simulink model "example1"  (R2024b)
settings: Solver=FixedStepAuto  StartTime=0.0  StopTime=20  FixedStep=0.001  RelTol=1e-3
(part 3 of 3)

== system example1/Subsystem15/SAT ==
  In1 : Inport
  Constant : Constant  Value=-1000
  Constant1 : Constant  Value=1000
  If : If  IfExpression=u1 < -1000  ElseIfExpressions=u1 > 1000
  If Action Subsystem : Subsystem  TreatAsAtomicUnit=on
  If Action Subsystem1 : Subsystem  TreatAsAtomicUnit=on
  If Action Subsystem2 : Subsystem  TreatAsAtomicUnit=on
  Merge : Merge  Inputs=3
  u1 : Outport
  wires:
  In1/1 -> If Action Subsystem1/1(In1), If/1
  If/1 -> If Action Subsystem/Action
  Constant/1 -> If Action Subsystem/1(In1)
  If/3 -> If Action Subsystem1/Action
  If/2 -> If Action Subsystem2/Action
  Constant1/1 -> If Action Subsystem2/1(In1)
  If Action Subsystem/1(Out1) -> Merge/1
  If Action Subsystem1/1(Out1) -> Merge/3
  If Action Subsystem2/1(Out1) -> Merge/2
  Merge/1 -> u1/1

== system example1/Subsystem15/Subsystem ==
  alpha : Inport
  Abs : Abs  SaturateOnIntegerOverflow=off
  Abs1 : Abs  SaturateOnIntegerOverflow=off
  Add : Sum  Inputs=+-
  Constant : Constant  Value=1/2
  Constant1 : Constant  Value=2/3
  Divide : Product  Inputs=*/
  Gain : Gain  Gain=-1
  Integrator : Integrator
  Integrator1 : Integrator
  Pow : Math  Operator=pow  SignedPower=on  RndMeth=Zero
  Pow1 : Math  Operator=pow  SignedPower=on  RndMeth=Zero
  Product{,1..3} (4 alike) : Product
  Product4 : Product  Inputs=3
  Sign : Signum
  Sign1 : Signum
  Sum : Sum  Inputs=|++
  k1 : Constant  Value=0.01
  k2 : Constant  Value=0.1
  xi : Constant
  tao1 : Outport
  tao2 : Outport  Port=2
  wires:
  alpha/1 -> Add/2
  Add/1 -> Pow/1, Sign/1
  Constant/1 -> Pow/2
  Pow/1 -> Abs/1
  Abs/1 -> Product/2
  Sign/1 -> Product/1
  Product/1 -> Product1/2
  k1/1 -> Product1/1
  Product1/1 -> Sum/1
  xi/1 -> Product4/2, Product4/3, Divide/2
  Divide/1 -> Sign1/1, Pow1/1
  Constant1/1 -> Pow1/2
  Pow1/1 -> Abs1/1
  Abs1/1 -> Product2/2
  Sign1/1 -> Product2/1
  Product2/1 -> Product3/1
  k2/1 -> Product3/2
  Product3/1 -> Sum/2
  Sum/1 -> Product4/1
  Product4/1 -> Gain/1
  Gain/1 -> Integrator/1
  Integrator/1 -> Divide/1, Integrator1/1, tao2/1
  Integrator1/1 -> Add/1, tao1/1

== system example1/Subsystem15/g22 ==
  x21 : Inport
  x22 : Inport  Port=2
  Constant : Constant  Value=4/5
  Sin : Trigonometry
  Sum : Sum  Inputs=|++
  Sum1 : Sum  Inputs=|++
  "[2]^1_1" : Subsystem
  g22 : Outport
  wires:
  x22/1 -> Sum1/2, "[2]^1_1"/2(2)
  Constant/1 -> "[2]^1_1"/1(In1)
  "[2]^1_1"/1(Out1) -> Sum/2
  Sum/1 -> g22/1
  x21/1 -> Sum1/1
  Sum1/1 -> Sin/1
  Sin/1 -> Sum/1

== system example1/Subsystem17/SAT ==
  In1 : Inport
  Constant : Constant  Value=-2000
  Constant1 : Constant  Value=2000
  If : If  IfExpression=u1 < -2000  ElseIfExpressions=u1 > 2000
  If Action Subsystem : Subsystem  TreatAsAtomicUnit=on
  If Action Subsystem1 : Subsystem  TreatAsAtomicUnit=on
  If Action Subsystem2 : Subsystem  TreatAsAtomicUnit=on
  Merge : Merge  Inputs=3
  u1 : Outport
  wires:
  In1/1 -> If Action Subsystem1/1(In1), If/1
  If/1 -> If Action Subsystem/Action
  Constant/1 -> If Action Subsystem/1(In1)
  If/3 -> If Action Subsystem1/Action
  If/2 -> If Action Subsystem2/Action
  Constant1/1 -> If Action Subsystem2/1(In1)
  If Action Subsystem/1(Out1) -> Merge/1
  If Action Subsystem1/1(Out1) -> Merge/3
  If Action Subsystem2/1(Out1) -> Merge/2
  Merge/1 -> u1/1

== system example1/Subsystem17/Subsystem ==
  alpha : Inport
  Abs : Abs  SaturateOnIntegerOverflow=off
  Abs1 : Abs  SaturateOnIntegerOverflow=off
  Add : Sum  Inputs=+-
  Constant : Constant  Value=1/2
  Constant1 : Constant  Value=2/3
  Divide : Product  Inputs=*/
  Gain : Gain  Gain=-1
  Integrator : Integrator
  Integrator1 : Integrator
  Pow : Math  Operator=pow  SignedPower=on  RndMeth=Zero
  Pow1 : Math  Operator=pow  SignedPower=on  RndMeth=Zero
  Product{,1..3} (4 alike) : Product
  Product4 : Product  Inputs=3
  Sign : Signum
  Sign1 : Signum
  Sum : Sum  Inputs=|++
  k1 : Constant  Value=0.01
  k2 : Constant  Value=0.1
  xi : Constant  Value=3
  tao1 : Outport
  tao2 : Outport  Port=2
  wires:
  alpha/1 -> Add/2
  Add/1 -> Pow/1, Sign/1
  Constant/1 -> Pow/2
  Pow/1 -> Abs/1
  Abs/1 -> Product/2
  Sign/1 -> Product/1
  Product/1 -> Product1/2
  k1/1 -> Product1/1
  Product1/1 -> Sum/1
  xi/1 -> Product4/2, Product4/3, Divide/2
  Divide/1 -> Sign1/1, Pow1/1
  Constant1/1 -> Pow1/2
  Pow1/1 -> Abs1/1
  Abs1/1 -> Product2/2
  Sign1/1 -> Product2/1
  Product2/1 -> Product3/1
  k2/1 -> Product3/2
  Product3/1 -> Sum/2
  Sum/1 -> Product4/1
  Product4/1 -> Gain/1
  Gain/1 -> Integrator/1
  Integrator/1 -> Divide/1, Integrator1/1, tao2/1
  Integrator1/1 -> Add/1, tao1/1

== system example1/Subsystem17/[2]^1_1 ==
  p/q : Inport
  2 : Inport  Port=2
  Abs : Abs  SaturateOnIntegerOverflow=off
  Pow : Math  Operator=pow  SignedPower=on  RndMeth=Zero
  Product : Product
  Sign : Signum
  Out1 : Outport
  wires:
  2/1 -> Sign/1, Abs/1
  Abs/1 -> Pow/1
  p/q/1 -> Pow/2
  Pow/1 -> Product/2
  Sign/1 -> Product/1
  Product/1 -> Out1/1

== system example1/Subsystem17/[2]^1_2 ==
  In1 : Inport
  2 : Inport  Port=2
  Abs : Abs  SaturateOnIntegerOverflow=off
  Pow : Math  Operator=pow  SignedPower=on  RndMeth=Zero
  Product : Product
  Sign : Signum
  Out1 : Outport
  wires:
  2/1 -> Sign/1, Abs/1
  Abs/1 -> Pow/1
  In1/1 -> Pow/2
  Pow/1 -> Product/2
  Sign/1 -> Product/1
  Product/1 -> Out1/1

== system example1/Subsystem17/g12 ==
  x11 : Inport
  x12 : Inport  Port=2
  Add : Sum  Inputs=3
  Cos : Trigonometry  Operator=cos
  Gain : Gain  Gain=0.01
  Product : Product
  Sin : Trigonometry
  Sin1 : Trigonometry
  g12 : Outport
  wires:
  x12/1 -> Product/2, Sin/1
  Add/1 -> g12/1
  x11/1 -> Product/1, Cos/1
  Cos/1 -> Add/1
  Product/1 -> Gain/1
  Gain/1 -> Sin1/1
  Sin1/1 -> Add/3
  Sin/1 -> Add/2

== system example1/Subsystem18/SAT ==
  In1 : Inport
  Constant : Constant  Value=-1000
  Constant1 : Constant  Value=1000
  If : If  IfExpression=u1 < -1000  ElseIfExpressions=u1 > 1000
  If Action Subsystem : Subsystem  TreatAsAtomicUnit=on
  If Action Subsystem1 : Subsystem  TreatAsAtomicUnit=on
  If Action Subsystem2 : Subsystem  TreatAsAtomicUnit=on
  Merge : Merge  Inputs=3
  u1 : Outport
  wires:
  In1/1 -> If Action Subsystem1/1(In1), If/1
  If/1 -> If Action Subsystem/Action
  Constant/1 -> If Action Subsystem/1(In1)
  If/3 -> If Action Subsystem1/Action
  If/2 -> If Action Subsystem2/Action
  Constant1/1 -> If Action Subsystem2/1(In1)
  If Action Subsystem/1(Out1) -> Merge/1
  If Action Subsystem1/1(Out1) -> Merge/3
  If Action Subsystem2/1(Out1) -> Merge/2
  Merge/1 -> u1/1

== system example1/Subsystem18/Subsystem ==
  alpha : Inport
  Abs : Abs  SaturateOnIntegerOverflow=off
  Abs1 : Abs  SaturateOnIntegerOverflow=off
  Add : Sum  Inputs=+-
  Constant : Constant  Value=1/2
  Constant1 : Constant  Value=2/3
  Divide : Product  Inputs=*/
  Gain : Gain  Gain=-1
  Integrator : Integrator
  Integrator1 : Integrator
  Pow : Math  Operator=pow  SignedPower=on  RndMeth=Zero
  Pow1 : Math  Operator=pow  SignedPower=on  RndMeth=Zero
  Product{,1..3} (4 alike) : Product
  Product4 : Product  Inputs=3
  Sign : Signum
  Sign1 : Signum
  Sum : Sum  Inputs=|++
  k1 : Constant  Value=0.01
  k2 : Constant  Value=0.1
  xi : Constant  Value=3
  tao1 : Outport
  tao2 : Outport  Port=2
  wires:
  alpha/1 -> Add/2
  Add/1 -> Pow/1, Sign/1
  Constant/1 -> Pow/2
  Pow/1 -> Abs/1
  Abs/1 -> Product/2
  Sign/1 -> Product/1
  Product/1 -> Product1/2
  k1/1 -> Product1/1
  Product1/1 -> Sum/1
  xi/1 -> Product4/2, Product4/3, Divide/2
  Divide/1 -> Sign1/1, Pow1/1
  Constant1/1 -> Pow1/2
  Pow1/1 -> Abs1/1
  Abs1/1 -> Product2/2
  Sign1/1 -> Product2/1
  Product2/1 -> Product3/1
  k2/1 -> Product3/2
  Product3/1 -> Sum/2
  Sum/1 -> Product4/1
  Product4/1 -> Gain/1
  Gain/1 -> Integrator/1
  Integrator/1 -> Divide/1, Integrator1/1, tao2/1
  Integrator1/1 -> Add/1, tao1/1

== system example1/Subsystem18/g22 ==
  x21 : Inport
  x22 : Inport  Port=2
  Constant : Constant  Value=4/5
  Sin : Trigonometry
  Sum : Sum  Inputs=|++
  Sum1 : Sum  Inputs=|++
  "[2]^1_1" : Subsystem
  g22 : Outport
  wires:
  x22/1 -> "[2]^1_1"/2(2)
  Constant/1 -> "[2]^1_1"/1(In1)
  "[2]^1_1"/1(Out1) -> Sum/2
  Sum/1 -> g22/1
  x21/1 -> Sum1/1
  Sum1/1 -> Sin/1
  Sin/1 -> Sum/1

== system example1/Subsystem24/SAT ==
  In1 : Inport
  Constant : Constant  Value=-1500
  Constant1 : Constant  Value=1500
  If : If  IfExpression=u1 < -1500  ElseIfExpressions=u1 > 1500
  If Action Subsystem : Subsystem  TreatAsAtomicUnit=on
  If Action Subsystem1 : Subsystem  TreatAsAtomicUnit=on
  If Action Subsystem2 : Subsystem  TreatAsAtomicUnit=on
  Merge : Merge  Inputs=3
  u1 : Outport
  wires:
  In1/1 -> If Action Subsystem1/1(In1), If/1
  If/1 -> If Action Subsystem/Action
  Constant/1 -> If Action Subsystem/1(In1)
  If/3 -> If Action Subsystem1/Action
  If/2 -> If Action Subsystem2/Action
  Constant1/1 -> If Action Subsystem2/1(In1)
  If Action Subsystem/1(Out1) -> Merge/1
  If Action Subsystem1/1(Out1) -> Merge/3
  If Action Subsystem2/1(Out1) -> Merge/2
  Merge/1 -> u1/1

== system example1/Subsystem24/Subsystem ==
  alpha : Inport
  Abs : Abs  SaturateOnIntegerOverflow=off
  Abs1 : Abs  SaturateOnIntegerOverflow=off
  Add : Sum  Inputs=+-
  Constant : Constant  Value=1/2
  Constant1 : Constant  Value=2/3
  Divide : Product  Inputs=*/
  Gain : Gain  Gain=-1
  Integrator : Integrator
  Integrator1 : Integrator
  Pow : Math  Operator=pow  SignedPower=on  RndMeth=Zero
  Pow1 : Math  Operator=pow  SignedPower=on  RndMeth=Zero
  Product{,1..3} (4 alike) : Product
  Product4 : Product  Inputs=3
  Sign : Signum
  Sign1 : Signum
  Sum : Sum  Inputs=|++
  k1 : Constant  Value=0.01
  k2 : Constant  Value=0.1
  xi : Constant  Value=3
  tao1 : Outport
  tao2 : Outport  Port=2
  wires:
  alpha/1 -> Add/2
  Add/1 -> Pow/1, Sign/1
  Constant/1 -> Pow/2
  Pow/1 -> Abs/1
  Abs/1 -> Product/2
  Sign/1 -> Product/1
  Product/1 -> Product1/2
  k1/1 -> Product1/1
  Product1/1 -> Sum/1
  xi/1 -> Product4/2, Product4/3, Divide/2
  Divide/1 -> Sign1/1, Pow1/1
  Constant1/1 -> Pow1/2
  Pow1/1 -> Abs1/1
  Abs1/1 -> Product2/2
  Sign1/1 -> Product2/1
  Product2/1 -> Product3/1
  k2/1 -> Product3/2
  Product3/1 -> Sum/2
  Sum/1 -> Product4/1
  Product4/1 -> Gain/1
  Gain/1 -> Integrator/1
  Integrator/1 -> Divide/1, Integrator1/1, tao2/1
  Integrator1/1 -> Add/1, tao1/1

== system example1/Subsystem24/[2]^1_1 ==
  In1 : Inport
  2 : Inport  Port=2
  Abs : Abs  SaturateOnIntegerOverflow=off
  Pow : Math  Operator=pow  SignedPower=on  RndMeth=Zero
  Product : Product
  Sign : Signum
  Out1 : Outport
  wires:
  2/1 -> Sign/1, Abs/1
  Abs/1 -> Pow/1
  In1/1 -> Pow/2
  Pow/1 -> Product/2
  Sign/1 -> Product/1
  Product/1 -> Out1/1

== system example1/Subsystem24/[2]^1_2 ==
  p/q : Inport
  2 : Inport  Port=2
  Abs : Abs  SaturateOnIntegerOverflow=off
  Pow : Math  Operator=pow  SignedPower=on  RndMeth=Zero
  Product : Product
  Sign : Signum
  Out1 : Outport
  wires:
  2/1 -> Sign/1, Abs/1
  Abs/1 -> Pow/1
  p/q/1 -> Pow/2
  Pow/1 -> Product/2
  Sign/1 -> Product/1
  Product/1 -> Out1/1

== system example1/Subsystem24/g12 ==
  x11 : Inport
  x12 : Inport  Port=2
  Cos : Trigonometry
  Sin : Trigonometry  Operator=cos
  Sum : Sum  Inputs=|++
  g12 : Outport
  wires:
  x12/1 -> Sin/1
  x11/1 -> Cos/1
  Cos/1 -> Sum/1
  Sin/1 -> Sum/2
  Sum/1 -> g12/1

== system example1/Subsystem9/SAT ==
  In1 : Inport
  Constant : Constant  Value=-1200
  Constant1 : Constant  Value=1200
  If : If  IfExpression=u1 < -1200  ElseIfExpressions=u1 > 1200
  If Action Subsystem : Subsystem  TreatAsAtomicUnit=on
  If Action Subsystem1 : Subsystem  TreatAsAtomicUnit=on
  If Action Subsystem2 : Subsystem  TreatAsAtomicUnit=on
  Merge : Merge  Inputs=3
  u1 : Outport
  wires:
  In1/1 -> If Action Subsystem1/1(In1), If/1
  If/1 -> If Action Subsystem/Action
  Constant/1 -> If Action Subsystem/1(In1)
  If/3 -> If Action Subsystem1/Action
  If/2 -> If Action Subsystem2/Action
  Constant1/1 -> If Action Subsystem2/1(In1)
  If Action Subsystem/1(Out1) -> Merge/1
  If Action Subsystem1/1(Out1) -> Merge/3
  If Action Subsystem2/1(Out1) -> Merge/2
  Merge/1 -> u1/1

== system example1/Subsystem9/Subsystem ==
  alpha : Inport
  Abs : Abs  SaturateOnIntegerOverflow=off
  Abs1 : Abs  SaturateOnIntegerOverflow=off
  Add : Sum  Inputs=+-
  Constant : Constant  Value=1/2
  Constant1 : Constant  Value=2/3
  Divide : Product  Inputs=*/
  Gain : Gain  Gain=-1
  Integrator : Integrator
  Integrator1 : Integrator
  Pow : Math  Operator=pow  SignedPower=on  RndMeth=Zero
  Pow1 : Math  Operator=pow  SignedPower=on  RndMeth=Zero
  Product{,1..3} (4 alike) : Product
  Product4 : Product  Inputs=3
  Sign : Signum
  Sign1 : Signum
  Sum : Sum  Inputs=|++
  k1 : Constant  Value=0.01
  k2 : Constant  Value=0.1
  xi : Constant
  tao1 : Outport
  tao2 : Outport  Port=2
  wires:
  alpha/1 -> Add/2
  Add/1 -> Pow/1, Sign/1
  Constant/1 -> Pow/2
  Pow/1 -> Abs/1
  Abs/1 -> Product/2
  Sign/1 -> Product/1
  Product/1 -> Product1/2
  k1/1 -> Product1/1
  Product1/1 -> Sum/1
  xi/1 -> Product4/2, Product4/3, Divide/2
  Divide/1 -> Sign1/1, Pow1/1
  Constant1/1 -> Pow1/2
  Pow1/1 -> Abs1/1
  Abs1/1 -> Product2/2
  Sign1/1 -> Product2/1
  Product2/1 -> Product3/1
  k2/1 -> Product3/2
  Product3/1 -> Sum/2
  Sum/1 -> Product4/1
  Product4/1 -> Gain/1
  Gain/1 -> Integrator/1
  Integrator/1 -> Divide/1, Integrator1/1, tao2/1
  Integrator1/1 -> Add/1, tao1/1

== system example1/Subsystem9/[2]^1_1 ==
  In1 : Inport
  2 : Inport  Port=2
  Abs : Abs  SaturateOnIntegerOverflow=off
  Pow : Math  Operator=pow  SignedPower=on  RndMeth=Zero
  Product : Product
  Sign : Signum
  Out1 : Outport
  wires:
  2/1 -> Sign/1, Abs/1
  Abs/1 -> Pow/1
  In1/1 -> Pow/2
  Pow/1 -> Product/2
  Sign/1 -> Product/1
  Product/1 -> Out1/1

== system example1/Subsystem9/[2]^1_2 ==
  p/q : Inport
  2 : Inport  Port=2
  Abs : Abs  SaturateOnIntegerOverflow=off
  Pow : Math  Operator=pow  SignedPower=on  RndMeth=Zero
  Product : Product
  Sign : Signum
  Out1 : Outport
  wires:
  2/1 -> Sign/1, Abs/1
  Abs/1 -> Pow/1
  p/q/1 -> Pow/2
  Pow/1 -> Product/2
  Sign/1 -> Product/1
  Product/1 -> Out1/1

== system example1/Subsystem9/g12 ==
  x11 : Inport
  x12 : Inport  Port=2
  Cos : Trigonometry  Operator=cos
  Sin : Trigonometry
  Sum : Sum  Inputs=|++
  g12 : Outport
  wires:
  x12/1 -> Sin/1
  x11/1 -> Cos/1
  Cos/1 -> Sum/1
  Sin/1 -> Sum/2
  Sum/1 -> g12/1

== system example1/alpha1/SAT ==
  In1 : Inport
  Constant : Constant  Value=-100
  Constant1 : Constant  Value=100
  If : If  IfExpression=u1 < -100  ElseIfExpressions=u1 > 100
  If Action Subsystem : Subsystem  TreatAsAtomicUnit=on
  If Action Subsystem1 : Subsystem  TreatAsAtomicUnit=on
  If Action Subsystem2 : Subsystem  TreatAsAtomicUnit=on
  Merge : Merge  Inputs=3
  u1 : Outport
  wires:
  In1/1 -> If Action Subsystem1/1(In1), If/1
  If/1 -> If Action Subsystem/Action
  Constant/1 -> If Action Subsystem/1(In1)
  If/3 -> If Action Subsystem1/Action
  If/2 -> If Action Subsystem2/Action
  Constant1/1 -> If Action Subsystem2/1(In1)
  If Action Subsystem/1(Out1) -> Merge/1
  If Action Subsystem1/1(Out1) -> Merge/3
  If Action Subsystem2/1(Out1) -> Merge/2
  Merge/1 -> u1/1

== system example1/alpha1/[2]^1_1 ==
  In1 : Inport
  2 : Inport  Port=2
  Abs : Abs  SaturateOnIntegerOverflow=off
  Pow : Math  Operator=pow  SignedPower=on  RndMeth=Zero
  Product : Product
  Sign : Signum
  Out1 : Outport
  wires:
  2/1 -> Sign/1, Abs/1
  Abs/1 -> Pow/1
  In1/1 -> Pow/2
  Pow/1 -> Product/2
  Sign/1 -> Product/1
  Product/1 -> Out1/1

== system example1/alpha1/[2]^1_2 ==
  p/q : Inport
  2 : Inport  Port=2
  Abs : Abs  SaturateOnIntegerOverflow=off
  Pow : Math  Operator=pow  SignedPower=on  RndMeth=Zero
  Product : Product
  Sign : Signum
  Out1 : Outport
  wires:
  2/1 -> Sign/1, Abs/1
  Abs/1 -> Pow/1
  p/q/1 -> Pow/2
  Pow/1 -> Product/2
  Sign/1 -> Product/1
  Product/1 -> Out1/1

== system example1/alpha1/g11 ==
  x11 : Inport
  Cos : Trigonometry  Operator=cos
  Sum : Sum  Inputs=|++
  g11 : Outport
  wires:
  Cos/1 -> Sum/1
  Sum/1 -> g11/1
  x11/1 -> Sum/2, Cos/1

== system example1/alpha2/[2]^1_1 ==
  p/q : Inport
  2 : Inport  Port=2
  Abs : Abs  SaturateOnIntegerOverflow=off
  Pow : Math  Operator=pow  SignedPower=on  RndMeth=Zero
  Product : Product
  Sign : Signum
  Out1 : Outport
  wires:
  2/1 -> Sign/1, Abs/1
  Abs/1 -> Pow/1
  p/q/1 -> Pow/2
  Pow/1 -> Product/2
  Sign/1 -> Product/1
  Product/1 -> Out1/1

== system example1/alpha2/[2]^1_2 ==
  In1 : Inport
  2 : Inport  Port=2
  Abs : Abs  SaturateOnIntegerOverflow=off
  Pow : Math  Operator=pow  SignedPower=on  RndMeth=Zero
  Product : Product
  Sign : Signum
  Out1 : Outport
  wires:
  2/1 -> Sign/1, Abs/1
  Abs/1 -> Pow/1
  In1/1 -> Pow/2
  Pow/1 -> Product/2
  Sign/1 -> Product/1
  Product/1 -> Out1/1

== system example1/alpha2/g21 ==
  x21 : Inport
  Cos : Trigonometry  Operator=cos
  Product : Product
  Sin : Trigonometry
  Sum : Sum  Inputs=|++
  g21 : Outport
  wires:
  x21/1 -> Cos/1, Sin/1, Sum/1
  Sum/1 -> g21/1
  Sin/1 -> Product/1
  Cos/1 -> Product/2
  Product/1 -> Sum/2

== system example1/alpha3/[2]^1_1 ==
  p/q : Inport
  2 : Inport  Port=2
  Abs : Abs  SaturateOnIntegerOverflow=off
  Pow : Math  Operator=pow  SignedPower=on  RndMeth=Zero
  Product : Product
  Sign : Signum
  Out1 : Outport
  wires:
  2/1 -> Sign/1, Abs/1
  Abs/1 -> Pow/1
  p/q/1 -> Pow/2
  Pow/1 -> Product/2
  Sign/1 -> Product/1
  Product/1 -> Out1/1

== system example1/alpha3/[2]^1_2 ==
  In1 : Inport
  2 : Inport  Port=2
  Abs : Abs  SaturateOnIntegerOverflow=off
  Pow : Math  Operator=pow  SignedPower=on  RndMeth=Zero
  Product : Product
  Sign : Signum
  Out1 : Outport
  wires:
  2/1 -> Sign/1, Abs/1
  Abs/1 -> Pow/1
  In1/1 -> Pow/2
  Pow/1 -> Product/2
  Sign/1 -> Product/1
  Product/1 -> Out1/1

== system example1/alpha3/g11 ==
  x11 : Inport
  Sin : Trigonometry
  g11 : Outport
  wires:
  Sin/1 -> g11/1
  x11/1 -> Sin/1

== system example1/alpha4/g21 ==
  x21 : Inport
  Cos : Trigonometry  Operator=cos
  Product : Product
  Product1 : Product
  Sin : Trigonometry
  g21 : Outport
  wires:
  x21/1 -> Cos/1, Sin/1
  Sin/1 -> Product/1
  Product/1 -> g21/1
  Cos/1 -> Product1/1, Product1/2
  Product1/1 -> Product/2

== system example1/alpha5/SAT ==
  In1 : Inport
  Constant : Constant  Value=-100
  Constant1 : Constant  Value=100
  If : If  IfExpression=u1 < -100  ElseIfExpressions=u1 > 100
  If Action Subsystem : Subsystem  TreatAsAtomicUnit=on
  If Action Subsystem1 : Subsystem  TreatAsAtomicUnit=on
  If Action Subsystem2 : Subsystem  TreatAsAtomicUnit=on
  Merge : Merge  Inputs=3
  u1 : Outport
  wires:
  In1/1 -> If Action Subsystem1/1(In1), If/1
  If/1 -> If Action Subsystem/Action
  Constant/1 -> If Action Subsystem/1(In1)
  If/3 -> If Action Subsystem1/Action
  If/2 -> If Action Subsystem2/Action
  Constant1/1 -> If Action Subsystem2/1(In1)
  If Action Subsystem/1(Out1) -> Merge/1
  If Action Subsystem1/1(Out1) -> Merge/3
  If Action Subsystem2/1(Out1) -> Merge/2
  Merge/1 -> u1/1

== system example1/alpha5/[2]^1_1 ==
  In1 : Inport
  2 : Inport  Port=2
  Abs : Abs  SaturateOnIntegerOverflow=off
  Pow : Math  Operator=pow  SignedPower=on  RndMeth=Zero
  Product : Product
  Sign : Signum
  Out1 : Outport
  wires:
  2/1 -> Sign/1, Abs/1
  Abs/1 -> Pow/1
  In1/1 -> Pow/2
  Pow/1 -> Product/2
  Sign/1 -> Product/1
  Product/1 -> Out1/1

== system example1/alpha5/[2]^1_2 ==
  p/q : Inport
  2 : Inport  Port=2
  Abs : Abs  SaturateOnIntegerOverflow=off
  Pow : Math  Operator=pow  SignedPower=on  RndMeth=Zero
  Product : Product
  Sign : Signum
  Out1 : Outport
  wires:
  2/1 -> Sign/1, Abs/1
  Abs/1 -> Pow/1
  p/q/1 -> Pow/2
  Pow/1 -> Product/2
  Sign/1 -> Product/1
  Product/1 -> Out1/1

== system example1/alpha5/g11 ==
  x11 : Inport
  Cos : Trigonometry
  Sum : Sum  Inputs=|++
  g11 : Outport
  wires:
  Cos/1 -> Sum/1
  Sum/1 -> g11/1
  x11/1 -> Sum/2, Cos/1

== system example1/alpha6/[2]^1_1 ==
  p/q : Inport
  2 : Inport  Port=2
  Abs : Abs  SaturateOnIntegerOverflow=off
  Pow : Math  Operator=pow  SignedPower=on  RndMeth=Zero
  Product : Product
  Sign : Signum
  Out1 : Outport
  wires:
  2/1 -> Sign/1, Abs/1
  Abs/1 -> Pow/1
  p/q/1 -> Pow/2
  Pow/1 -> Product/2
  Sign/1 -> Product/1
  Product/1 -> Out1/1

== system example1/alpha6/[2]^1_2 ==
  In1 : Inport
  2 : Inport  Port=2
  Abs : Abs  SaturateOnIntegerOverflow=off
  Pow : Math  Operator=pow  SignedPower=on  RndMeth=Zero
  Product : Product
  Sign : Signum
  Out1 : Outport
  wires:
  2/1 -> Sign/1, Abs/1
  Abs/1 -> Pow/1
  In1/1 -> Pow/2
  Pow/1 -> Product/2
  Sign/1 -> Product/1
  Product/1 -> Out1/1

== system example1/alpha6/g21 ==
  x21 : Inport
  Cos : Trigonometry  Operator=cos
  Product : Product
  Sin : Trigonometry  Operator=cos
  Sum : Sum  Inputs=|++
  g21 : Outport
  wires:
  x21/1 -> Cos/1, Sin/1, Sum/1
  Sum/1 -> g21/1
  Sin/1 -> Product/1
  Cos/1 -> Product/2
  Product/1 -> Sum/2

== system example1/alpha7/[2]^1_1 ==
  p/q : Inport
  2 : Inport  Port=2
  Abs : Abs  SaturateOnIntegerOverflow=off
  Pow : Math  Operator=pow  SignedPower=on  RndMeth=Zero
  Product : Product
  Sign : Signum
  Out1 : Outport
  wires:
  2/1 -> Sign/1, Abs/1
  Abs/1 -> Pow/1
  p/q/1 -> Pow/2
  Pow/1 -> Product/2
  Sign/1 -> Product/1
  Product/1 -> Out1/1

== system example1/alpha7/[2]^1_2 ==
  In1 : Inport
  2 : Inport  Port=2
  Abs : Abs  SaturateOnIntegerOverflow=off
  Pow : Math  Operator=pow  SignedPower=on  RndMeth=Zero
  Product : Product
  Sign : Signum
  Out1 : Outport
  wires:
  2/1 -> Sign/1, Abs/1
  Abs/1 -> Pow/1
  In1/1 -> Pow/2
  Pow/1 -> Product/2
  Sign/1 -> Product/1
  Product/1 -> Out1/1

== system example1/alpha7/g11 ==
  x11 : Inport
  Sin : Trigonometry  Operator=cos
  g11 : Outport
  wires:
  Sin/1 -> g11/1
  x11/1 -> Sin/1

== system example1/alpha8/g21 ==
  x21 : Inport
  Cos : Trigonometry  Operator=cos
  Product : Product
  Sin : Trigonometry
  g21 : Outport
  wires:
  x21/1 -> Cos/1, Sin/1
  Sin/1 -> Product/1
  Product/1 -> g21/1
  Cos/1 -> Product/2

== system example1/j-i_1/[2]^1_1 ==
  In1 : Inport
  2 : Inport  Port=2
  Abs : Abs  SaturateOnIntegerOverflow=off
  Pow : Math  Operator=pow  SignedPower=on  RndMeth=Zero
  Product : Product
  Sign : Signum
  Out1 : Outport
  wires:
  2/1 -> Sign/1, Abs/1
  Abs/1 -> Pow/1
  In1/1 -> Pow/2
  Pow/1 -> Product/2
  Sign/1 -> Product/1
  Product/1 -> Out1/1

== system example1/j-i_1/[2]^1_2 ==
  In1 : Inport
  2 : Inport  Port=2
  Abs : Abs  SaturateOnIntegerOverflow=off
  Pow : Math  Operator=pow  SignedPower=on  RndMeth=Zero
  Product : Product
  Sign : Signum
  Out1 : Outport
  wires:
  2/1 -> Sign/1, Abs/1
  Abs/1 -> Pow/1
  In1/1 -> Pow/2
  Pow/1 -> Product/2
  Sign/1 -> Product/1
  Product/1 -> Out1/1

== system example1/j-i_1/[2]^1_3 ==
  p/q : Inport
  2 : Inport  Port=2
  Abs : Abs  SaturateOnIntegerOverflow=off
  Pow : Math  Operator=pow  SignedPower=on  RndMeth=Zero
  Product : Product
  Sign : Signum
  Out1 : Outport
  wires:
  2/1 -> Sign/1, Abs/1
  Abs/1 -> Pow/1
  p/q/1 -> Pow/2
  Pow/1 -> Product/2
  Sign/1 -> Product/1
  Product/1 -> Out1/1

== system example1/j-i_1/[2]^1_4 ==
  In1 : Inport
  2 : Inport  Port=2
  Abs : Abs  SaturateOnIntegerOverflow=off
  Pow : Math  Operator=pow  SignedPower=on  RndMeth=Zero
  Product : Product
  Sign : Signum
  Out1 : Outport
  wires:
  2/1 -> Sign/1, Abs/1
  Abs/1 -> Pow/1
  In1/1 -> Pow/2
  Pow/1 -> Product/2
  Sign/1 -> Product/1
  Product/1 -> Out1/1

== system example1/j-i_2/[2]^1_1 ==
  In1 : Inport
  2 : Inport  Port=2
  Abs : Abs  SaturateOnIntegerOverflow=off
  Pow : Math  Operator=pow  SignedPower=on  RndMeth=Zero
  Product : Product
  Sign : Signum
  Out1 : Outport
  wires:
  2/1 -> Sign/1, Abs/1
  Abs/1 -> Pow/1
  In1/1 -> Pow/2
  Pow/1 -> Product/2
  Sign/1 -> Product/1
  Product/1 -> Out1/1

== system example1/j-i_2/[2]^1_2 ==
  In1 : Inport
  2 : Inport  Port=2
  Abs : Abs  SaturateOnIntegerOverflow=off
  Pow : Math  Operator=pow  SignedPower=on  RndMeth=Zero
  Product : Product
  Sign : Signum
  Out1 : Outport
  wires:
  2/1 -> Sign/1, Abs/1
  Abs/1 -> Pow/1
  In1/1 -> Pow/2
  Pow/1 -> Product/2
  Sign/1 -> Product/1
  Product/1 -> Out1/1

== system example1/j-i_2/[2]^1_3 ==
  In1 : Inport
  2 : Inport  Port=2
  Abs : Abs  SaturateOnIntegerOverflow=off
  Pow : Math  Operator=pow  SignedPower=on  RndMeth=Zero
  Product : Product
  Sign : Signum
  Out1 : Outport
  wires:
  2/1 -> Sign/1, Abs/1
  Abs/1 -> Pow/1
  In1/1 -> Pow/2
  Pow/1 -> Product/2
  Sign/1 -> Product/1
  Product/1 -> Out1/1

== system example1/j-i_2/[2]^1_4 ==
  In1 : Inport
  2 : Inport  Port=2
  Abs : Abs  SaturateOnIntegerOverflow=off
  Pow : Math  Operator=pow  SignedPower=on  RndMeth=Zero
  Product : Product
  Sign : Signum
  Out1 : Outport
  wires:
  2/1 -> Sign/1, Abs/1
  Abs/1 -> Pow/1
  In1/1 -> Pow/2
  Pow/1 -> Product/2
  Sign/1 -> Product/1
  Product/1 -> Out1/1

== system example1/j-i_5/[2]^1_1 ==
  In1 : Inport
  2 : Inport  Port=2
  Abs : Abs  SaturateOnIntegerOverflow=off
  Pow : Math  Operator=pow  SignedPower=on  RndMeth=Zero
  Product : Product
  Sign : Signum
  Out1 : Outport
  wires:
  2/1 -> Sign/1, Abs/1
  Abs/1 -> Pow/1
  In1/1 -> Pow/2
  Pow/1 -> Product/2
  Sign/1 -> Product/1
  Product/1 -> Out1/1

== system example1/j-i_5/[2]^1_2 ==
  In1 : Inport
  2 : Inport  Port=2
  Abs : Abs  SaturateOnIntegerOverflow=off
  Pow : Math  Operator=pow  SignedPower=on  RndMeth=Zero
  Product : Product
  Sign : Signum
  Out1 : Outport
  wires:
  2/1 -> Sign/1, Abs/1
  Abs/1 -> Pow/1
  In1/1 -> Pow/2
  Pow/1 -> Product/2
  Sign/1 -> Product/1
  Product/1 -> Out1/1

== system example1/j-i_5/[2]^1_3 ==
  p/q : Inport
  2 : Inport  Port=2
  Abs : Abs  SaturateOnIntegerOverflow=off
  Pow : Math  Operator=pow  SignedPower=on  RndMeth=Zero
  Product : Product
  Sign : Signum
  Out1 : Outport
  wires:
  2/1 -> Sign/1, Abs/1
  Abs/1 -> Pow/1
  p/q/1 -> Pow/2
  Pow/1 -> Product/2
  Sign/1 -> Product/1
  Product/1 -> Out1/1

== system example1/j-i_5/[2]^1_4 ==
  In1 : Inport
  2 : Inport  Port=2
  Abs : Abs  SaturateOnIntegerOverflow=off
  Pow : Math  Operator=pow  SignedPower=on  RndMeth=Zero
  Product : Product
  Sign : Signum
  Out1 : Outport
  wires:
  2/1 -> Sign/1, Abs/1
  Abs/1 -> Pow/1
  In1/1 -> Pow/2
  Pow/1 -> Product/2
  Sign/1 -> Product/1
  Product/1 -> Out1/1

== system example1/j-i_6/[2]^1_1 ==
  In1 : Inport
  2 : Inport  Port=2
  Abs : Abs  SaturateOnIntegerOverflow=off
  Pow : Math  Operator=pow  SignedPower=on  RndMeth=Zero
  Product : Product
  Sign : Signum
  Out1 : Outport
  wires:
  2/1 -> Sign/1, Abs/1
  Abs/1 -> Pow/1
  In1/1 -> Pow/2
  Pow/1 -> Product/2
  Sign/1 -> Product/1
  Product/1 -> Out1/1

== system example1/j-i_6/[2]^1_2 ==
  In1 : Inport
  2 : Inport  Port=2
  Abs : Abs  SaturateOnIntegerOverflow=off
  Pow : Math  Operator=pow  SignedPower=on  RndMeth=Zero
  Product : Product
  Sign : Signum
  Out1 : Outport
  wires:
  2/1 -> Sign/1, Abs/1
  Abs/1 -> Pow/1
  In1/1 -> Pow/2
  Pow/1 -> Product/2
  Sign/1 -> Product/1
  Product/1 -> Out1/1

== system example1/j-i_6/[2]^1_3 ==
  In1 : Inport
  2 : Inport  Port=2
  Abs : Abs  SaturateOnIntegerOverflow=off
  Pow : Math  Operator=pow  SignedPower=on  RndMeth=Zero
  Product : Product
  Sign : Signum
  Out1 : Outport
  wires:
  2/1 -> Sign/1, Abs/1
  Abs/1 -> Pow/1
  In1/1 -> Pow/2
  Pow/1 -> Product/2
  Sign/1 -> Product/1
  Product/1 -> Out1/1

== system example1/j-i_6/[2]^1_4 ==
  In1 : Inport
  2 : Inport  Port=2
  Abs : Abs  SaturateOnIntegerOverflow=off
  Pow : Math  Operator=pow  SignedPower=on  RndMeth=Zero
  Product : Product
  Sign : Signum
  Out1 : Outport
  wires:
  2/1 -> Sign/1, Abs/1
  Abs/1 -> Pow/1
  In1/1 -> Pow/2
  Pow/1 -> Product/2
  Sign/1 -> Product/1
  Product/1 -> Out1/1

== system example1/ESTIMAT4/g22/[2]^1_1 ==
  In1 : Inport
  2 : Inport  Port=2
  Abs : Abs  SaturateOnIntegerOverflow=off
  Pow : Math  Operator=pow  SignedPower=on  RndMeth=Zero
  Product : Product
  Sign : Signum
  Out1 : Outport
  wires:
  2/1 -> Sign/1, Abs/1
  Abs/1 -> Pow/1
  In1/1 -> Pow/2
  Pow/1 -> Product/2
  Sign/1 -> Product/1
  Product/1 -> Out1/1

== system example1/ESTIMAT7/g22/[2]^1_1 ==
  In1 : Inport
  2 : Inport  Port=2
  Abs : Abs  SaturateOnIntegerOverflow=off
  Pow : Math  Operator=pow  SignedPower=on  RndMeth=Zero
  Product : Product
  Sign : Signum
  Out1 : Outport
  wires:
  2/1 -> Sign/1, Abs/1
  Abs/1 -> Pow/1
  In1/1 -> Pow/2
  Pow/1 -> Product/2
  Sign/1 -> Product/1
  Product/1 -> Out1/1

== system example1/SYSTEM4/g22/[2]^1_1 ==
  In1 : Inport
  2 : Inport  Port=2
  Abs : Abs  SaturateOnIntegerOverflow=off
  Pow : Math  Operator=pow  SignedPower=on  RndMeth=Zero
  Product : Product
  Sign : Signum
  Out1 : Outport
  wires:
  2/1 -> Sign/1, Abs/1
  Abs/1 -> Pow/1
  In1/1 -> Pow/2
  Pow/1 -> Product/2
  Sign/1 -> Product/1
  Product/1 -> Out1/1

== system example1/SYSTEM8/g22/[2]^1_1 ==
  In1 : Inport
  2 : Inport  Port=2
  Abs : Abs  SaturateOnIntegerOverflow=off
  Pow : Math  Operator=pow  SignedPower=on  RndMeth=Zero
  Product : Product
  Sign : Signum
  Out1 : Outport
  wires:
  2/1 -> Sign/1, Abs/1
  Abs/1 -> Pow/1
  In1/1 -> Pow/2
  Pow/1 -> Product/2
  Sign/1 -> Product/1
  Product/1 -> Out1/1

== system example1/Subsystem1/SAT/If Action Subsystem ==
  In1 : Inport
  Action Port : ActionPort  ActionPortLabel=if(u1 < -2000)
  Out1 : Outport
  wires:
  In1/1 -> Out1/1

== system example1/Subsystem1/SAT/If Action Subsystem1 ==
  In1 : Inport
  Action Port : ActionPort  ActionPortLabel=else
  Out1 : Outport
  wires:
  In1/1 -> Out1/1

== system example1/Subsystem1/SAT/If Action Subsystem2 ==
  In1 : Inport
  Action Port : ActionPort  ActionPortLabel=elseif(u1 > 2000)
  Out1 : Outport
  wires:
  In1/1 -> Out1/1

== system example1/Subsystem10/SAT/If Action Subsystem ==
  In1 : Inport
  Action Port : ActionPort  ActionPortLabel=if(u1 < -1000)
  Out1 : Outport
  wires:
  In1/1 -> Out1/1

== system example1/Subsystem10/SAT/If Action Subsystem1 ==
  In1 : Inport
  Action Port : ActionPort  ActionPortLabel=else
  Out1 : Outport
  wires:
  In1/1 -> Out1/1

== system example1/Subsystem10/SAT/If Action Subsystem2 ==
  In1 : Inport
  Action Port : ActionPort  ActionPortLabel=elseif(u1 > 1000)
  Out1 : Outport
  wires:
  In1/1 -> Out1/1

== system example1/Subsystem14/SAT/If Action Subsystem ==
  In1 : Inport
  Action Port : ActionPort  ActionPortLabel=if(u1 < -1000)
  Out1 : Outport
  wires:
  In1/1 -> Out1/1

== system example1/Subsystem14/SAT/If Action Subsystem1 ==
  In1 : Inport
  Action Port : ActionPort  ActionPortLabel=else
  Out1 : Outport
  wires:
  In1/1 -> Out1/1

== system example1/Subsystem14/SAT/If Action Subsystem2 ==
  In1 : Inport
  Action Port : ActionPort  ActionPortLabel=elseif(u1 > 1000)
  Out1 : Outport
  wires:
  In1/1 -> Out1/1

== system example1/Subsystem15/SAT/If Action Subsystem ==
  In1 : Inport
  Action Port : ActionPort  ActionPortLabel=if(u1 < -1000)
  Out1 : Outport
  wires:
  In1/1 -> Out1/1

== system example1/Subsystem15/SAT/If Action Subsystem1 ==
  In1 : Inport
  Action Port : ActionPort  ActionPortLabel=else
  Out1 : Outport
  wires:
  In1/1 -> Out1/1

== system example1/Subsystem15/SAT/If Action Subsystem2 ==
  In1 : Inport
  Action Port : ActionPort  ActionPortLabel=elseif(u1 > 1000)
  Out1 : Outport
  wires:
  In1/1 -> Out1/1

== system example1/Subsystem15/g22/[2]^1_1 ==
  In1 : Inport
  2 : Inport  Port=2
  Abs : Abs  SaturateOnIntegerOverflow=off
  Pow : Math  Operator=pow  SignedPower=on  RndMeth=Zero
  Product : Product
  Sign : Signum
  Out1 : Outport
  wires:
  2/1 -> Sign/1, Abs/1
  Abs/1 -> Pow/1
  In1/1 -> Pow/2
  Pow/1 -> Product/2
  Sign/1 -> Product/1
  Product/1 -> Out1/1

== system example1/Subsystem17/SAT/If Action Subsystem ==
  In1 : Inport
  Action Port : ActionPort  ActionPortLabel=if(u1 < -2000)
  Out1 : Outport
  wires:
  In1/1 -> Out1/1

== system example1/Subsystem17/SAT/If Action Subsystem1 ==
  In1 : Inport
  Action Port : ActionPort  ActionPortLabel=else
  Out1 : Outport
  wires:
  In1/1 -> Out1/1

== system example1/Subsystem17/SAT/If Action Subsystem2 ==
  In1 : Inport
  Action Port : ActionPort  ActionPortLabel=elseif(u1 > 2000)
  Out1 : Outport
  wires:
  In1/1 -> Out1/1

== system example1/Subsystem18/SAT/If Action Subsystem ==
  In1 : Inport
  Action Port : ActionPort  ActionPortLabel=if(u1 < -1000)
  Out1 : Outport
  wires:
  In1/1 -> Out1/1

== system example1/Subsystem18/SAT/If Action Subsystem1 ==
  In1 : Inport
  Action Port : ActionPort  ActionPortLabel=else
  Out1 : Outport
  wires:
  In1/1 -> Out1/1

== system example1/Subsystem18/SAT/If Action Subsystem2 ==
  In1 : Inport
  Action Port : ActionPort  ActionPortLabel=elseif(u1 > 1000)
  Out1 : Outport
  wires:
  In1/1 -> Out1/1

== system example1/Subsystem18/g22/[2]^1_1 ==
  In1 : Inport
  2 : Inport  Port=2
  Abs : Abs  SaturateOnIntegerOverflow=off
  Pow : Math  Operator=pow  SignedPower=on  RndMeth=Zero
  Product : Product
  Sign : Signum
  Out1 : Outport
  wires:
  2/1 -> Sign/1, Abs/1
  Abs/1 -> Pow/1
  In1/1 -> Pow/2
  Pow/1 -> Product/2
  Sign/1 -> Product/1
  Product/1 -> Out1/1

== system example1/Subsystem24/SAT/If Action Subsystem ==
  In1 : Inport
  Action Port : ActionPort  ActionPortLabel=if(u1 < -1500)
  Out1 : Outport
  wires:
  In1/1 -> Out1/1

== system example1/Subsystem24/SAT/If Action Subsystem1 ==
  In1 : Inport
  Action Port : ActionPort  ActionPortLabel=else
  Out1 : Outport
  wires:
  In1/1 -> Out1/1

== system example1/Subsystem24/SAT/If Action Subsystem2 ==
  In1 : Inport
  Action Port : ActionPort  ActionPortLabel=elseif(u1 > 1500)
  Out1 : Outport
  wires:
  In1/1 -> Out1/1

== system example1/Subsystem9/SAT/If Action Subsystem ==
  In1 : Inport
  Action Port : ActionPort  ActionPortLabel=if(u1 < -1200)
  Out1 : Outport
  wires:
  In1/1 -> Out1/1

== system example1/Subsystem9/SAT/If Action Subsystem1 ==
  In1 : Inport
  Action Port : ActionPort  ActionPortLabel=else
  Out1 : Outport
  wires:
  In1/1 -> Out1/1

== system example1/Subsystem9/SAT/If Action Subsystem2 ==
  In1 : Inport
  Action Port : ActionPort  ActionPortLabel=elseif(u1 > 1200)
  Out1 : Outport
  wires:
  In1/1 -> Out1/1

== system example1/alpha1/SAT/If Action Subsystem ==
  In1 : Inport
  Action Port : ActionPort  ActionPortLabel=if(u1 < -100)
  Out1 : Outport
  wires:
  In1/1 -> Out1/1

== system example1/alpha1/SAT/If Action Subsystem1 ==
  In1 : Inport
  Action Port : ActionPort  ActionPortLabel=else
  Out1 : Outport
  wires:
  In1/1 -> Out1/1

== system example1/alpha1/SAT/If Action Subsystem2 ==
  In1 : Inport
  Action Port : ActionPort  ActionPortLabel=elseif(u1 > 100)
  Out1 : Outport
  wires:
  In1/1 -> Out1/1

== system example1/alpha5/SAT/If Action Subsystem ==
  In1 : Inport
  Action Port : ActionPort
  Out1 : Outport
  wires:
  In1/1 -> Out1/1

== system example1/alpha5/SAT/If Action Subsystem1 ==
  In1 : Inport
  Action Port : ActionPort
  Out1 : Outport
  wires:
  In1/1 -> Out1/1

== system example1/alpha5/SAT/If Action Subsystem2 ==
  In1 : Inport
  Action Port : ActionPort
  Out1 : Outport
  wires:
  In1/1 -> Out1/1
